simulink model "SDRE_MPTA_SDRE_newMODEL"  (R2024a)
settings: Solver=ode23t  StartTime=0  StopTime=27.8  RelTol=1e-3
values from neighbouring files (symbols this model uses):
  B = 0.002277    [initial_value.m]
  coef = readmatrix(ReadPath_coef)    [inital.m]
  command_t = readmatrix(ReadPath_command_t)    [inital.m]
  J = 0.00782    [initial_value.m]
  Lambda_m = 0.30175    [initial_value.m]
  Ld = 18e-3    (= 0.018)    [initial_value.m]
  Ldq = Ld - Lq    [inital.m]
  Lq = 32e-3    (= 0.032)    [initial_value.m]
  Polepairs = 3    [initial_value.m]
  rate1 = 3    [inital.m]
  rate2 = 1    [inital.m]
  Rs = 2.5    [initial_value.m]
  timestep = 1e-5    (= 1e-05)    [inital.m]
  V = [V_11 V_12;V_21 V_22]    [Create_MVG.m]
undefined symbols (not defined in the file or in its folder): rate
libraries: spsControlledVoltageSourceLib x6, spsPermanentMagnetSynchronousMachineLib x2, spsGroundLib x2, sps_lib x1
(part 1 of 2)
settings Model: Creator=User  LastModifiedBy=User

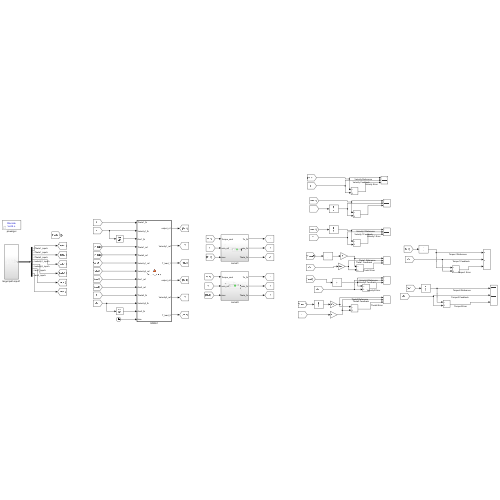
[thumbnail: Simulink's stored preview of the top-level diagram]
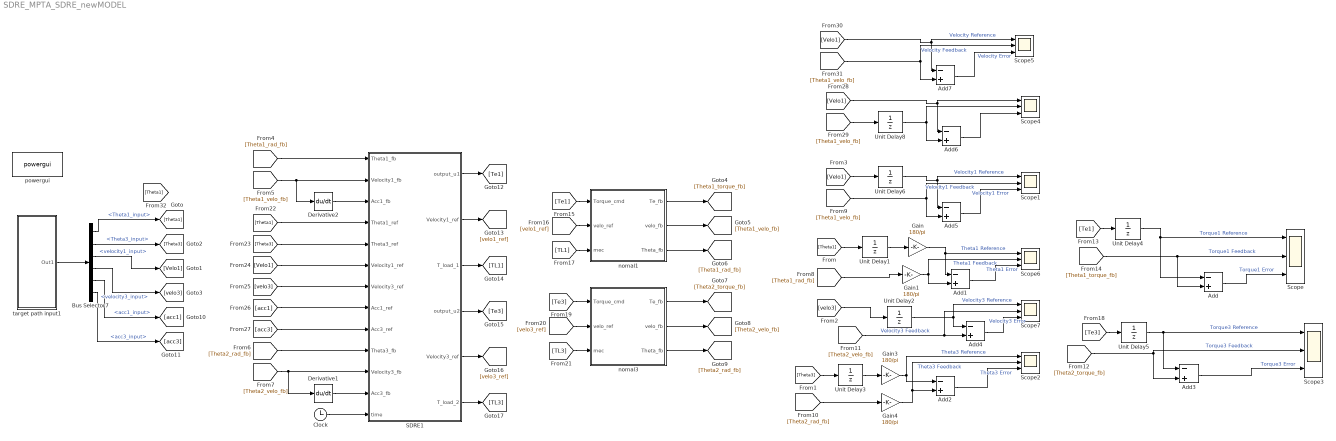
== system SDRE_MPTA_SDRE_newMODEL ==
  Add{,1..7} (8 alike) : Sum  Inputs=-+
  Bus Selector7 : BusSelector  OutputSignals=Theta1_input,Theta3_input,velocity1_input,velocity3_input,acc1_input,acc3_input
  Clock : Clock
  Derivative1 : Derivative
  Derivative2 : Derivative
  Gain{,1,3..4} (4 alike) : Gain  Gain=180/pi
  SDRE1 : MATLAB Function  TreatAsAtomicUnit=on
  Scope{,1..7} (8 alike) : Scope  NumInputPorts=3
  Unit Delay{1..6,8} (7 alike) : UnitDelay  SampleTime=1e-5  HasFrameUpgradeWarning=on
  nomal1 : Subsystem
  nomal3 : Subsystem
  powergui : sps_lib/powergui  Priority=1  SimulationMode=Discrete  SampleTime=timestep  frequency=60  Iterations=50  frequencyindice=0  Pbase=100e6  ErrMax=1e-4  UnitsV=kV  UnitsW=MW  buscounter=0  FunctionMessages=off  echomessages=off  EnableUseOfTLC=off  CurrentSourceSwitches=off  DisableSnubberDevices=off  DisableRonSwitches=off  DisableVfSwitches=off  DisplayEquations=off  AutomaticDiscreteSolvers=off  SolverType=Tustin/Backward Euler (TBE)  Interpol=off  ExternalGateDelay=off  methode=off  Ts=100  x0status=blocks  SPID=on  SwTol=0  HookPort=off  NonlinearTolerance=1e-4  nMaxIteration=100  ContinueOnMaxIteration=off  RestoreLinks=warning  ResistiveCurrentMeasurement=off  Frange=[0:2:500]  Ylog=off  Xlog=on  ShowGrid=off  save=off  variable=ZData  structure=0  ZoomFFT=off  StartTime=0.0  cycles=1  DisplayStyle=1  fundamental=60  FreqAxis=off  MaxFrequency=1000  frequencyindicesteady=1  RmsSteady=1  display=off
  target path input1 : Subsystem
  wires:
  Bus Selector7/4 -> [velo3]  "<velocity3_input>"
  Bus Selector7/2 -> [Theta3]  "<Theta3_input>"
  Bus Selector7/1 -> [Theta1]  "<Theta1_input>"
  Bus Selector7/3 -> [Velo1]  "<velocity1_input>"
  SDRE1/4(output_u2) -> [Te3]
  SDRE1/2(Velocity1_ref) -> [velo1_ref]
  [Theta3] -> Unit Delay3/1
  [velo3] -> Unit Delay2/1
  target path input1/1(Out1) -> Bus Selector7/1
  nomal1/1(Te_fb) -> [Theta1_torque_fb]
  nomal1/2(velo_fb) -> [Theta1_velo_fb]
  nomal1/3(Theta_fb) -> [Theta1_rad_fb]
  [Theta1_rad_fb] -> SDRE1/1(Theta1_fb)
  [Theta1_velo_fb] -> Derivative2/1, SDRE1/2(Velocity1_fb)
  [Theta2_rad_fb] -> SDRE1/10(Theta3_fb)
  [Theta2_velo_fb] -> Derivative1/1, SDRE1/11(Velocity3_fb)
  Gain/1 -> Add1/1, Scope6/1  "Theta1 Reference"
  Gain1/1 -> Scope6/2, Add1/2  "Theta1 Feedback"
  Gain3/1 -> Add2/1, Scope2/1  "Theta3 Reference"
  Gain4/1 -> Add2/2, Scope2/2  "Theta3 Feedback"
  Add2/1 -> Scope2/3  "Theta3 Error"
  Add1/1 -> Scope6/3  "Theta1 Error"
  Add3/1 -> Scope3/3  "Torque3 Error"
  Derivative1/1 -> SDRE1/12(Acc3_fb)
  Derivative2/1 -> SDRE1/3(Acc1_fb)
  Add/1 -> Scope/3  "Torque1 Error"
  Add4/1 -> Scope7/3  "Velocity3 Error"
  Add5/1 -> Scope1/3  "Velocity1 Error"
  Clock/1 -> SDRE1/13(time)
  SDRE1/1(output_u1) -> [Te1]
  [Theta1] -> Unit Delay1/1
  [Velo1] -> Unit Delay6/1
  [Theta2_velo_fb] -> Add4/2, Scope7/2  "Velocity3 Feedback"
  [Theta2_rad_fb] -> Gain4/1
  nomal3/3(Theta_fb) -> [Theta2_rad_fb]
  nomal3/2(velo_fb) -> [Theta2_velo_fb]
  nomal3/1(Te_fb) -> [Theta2_torque_fb]
  Bus Selector7/5 -> [acc1]  "<acc1_input>"
  Bus Selector7/6 -> [acc3]  "<acc3_input>"
  [Te1] -> Unit Delay4/1
  [Te1] -> nomal1/1(Torque_cmd)
  [velo1_ref] -> nomal1/2(velo_ref)
  SDRE1/3(T_load_1) -> [TL1]
  [TL1] -> nomal1/3(mec)
  [Te3] -> Unit Delay5/1
  SDRE1/5(Velocity3_ref) -> [velo3_ref]
  SDRE1/6(T_load_2) -> [TL3]
  [Te3] -> nomal3/1(Torque_cmd)
  [velo3_ref] -> nomal3/2(velo_ref)
  [TL3] -> nomal3/3(mec)
  [Theta1] -> SDRE1/4(Theta1_ref)
  [Theta3] -> SDRE1/5(Theta3_ref)
  [Velo1] -> SDRE1/6("Velocity1_ref ")
  [velo3] -> SDRE1/7("Velocity3_ref ")
  [acc1] -> SDRE1/8(Acc1_ref)
  [acc3] -> SDRE1/9(Acc3_ref)
  [Theta1_rad_fb] -> Gain1/1
  [Theta1_velo_fb] -> Add5/2, Scope1/2  "Velocity1 Feedback"
  [Theta1_torque_fb] -> Add/2, Scope/2  "Torque1 Feedback"
  [Theta2_torque_fb] -> Scope3/2, Add3/2  "Torque3 Feedback"
  Unit Delay6/1 -> Add5/1, Scope1/1  "Velocity1 Reference"
  Unit Delay1/1 -> Gain/1
  Unit Delay3/1 -> Gain3/1
  Unit Delay2/1 -> Scope7/1, Add4/1  "Velocity3 Reference"
  Unit Delay4/1 -> Add/1, Scope/1  "Torque1 Reference"
  Unit Delay5/1 -> Scope3/1, Add3/1  "Torque3 Reference"
  Add6/1 -> Scope4/3
  [Theta1_velo_fb] -> Unit Delay8/1
  [Velo1] -> Add6/1, Scope4/1
  Unit Delay8/1 -> Add6/2, Scope4/2
  Add7/1 -> Scope5/3  "Velocity Error"
  [Theta1_velo_fb] -> Add7/2, Scope5/2  "Velocity Feedback"
  [Velo1] -> Add7/1, Scope5/1  "Velocity Reference"

== system SDRE_MPTA_SDRE_newMODEL/nomal1 ==
  Torque_cmd : Inport
  velo_ref : Inport  Port=2
  mec : Inport  Port=3
  Constant2 : Constant  Value=Polepairs
  MTPA : MATLAB Function  TreatAsAtomicUnit=on
  Measure : Subsystem
  "Permanent Magnet Synchronous Machine " : spsPermanentMagnetSynchronousMachineLib/Permanent Magnet Synchronous Machine  NbPhases=3  FluxDistribution=Sinusoidal  RotorType=Salient-pole  MechanicalLoad=Torque Tm  PresetModel=No  ShowDetailedParameters=on  MeasurementBus=off  Resistance=Rs  Inductance=8.5e-3  dqInductances=[Ld Lq]  La=5.7e-3  MachineConstant=Flux linkage established by magnets (V.s)  Flux=Lambda_m  VoltageCst=164.1942  TorqueCst=1.3579  Flat=120  Mechanical=[J B Polepairs]  PolePairs=4  InitialConditions=[0,0, 0,0]  InitialConditions5ph=[0 0 0 0 0 0]  RefAngle=Aligned with phase A axis (original Park)  IterativeDiscreteModel=Trapezoidal non iterative  TsBlock=-1  TsPowergui=0
  Product1 : Product
  Unit Delay1 : UnitDelay  SampleTime=1e-5  HasFrameUpgradeWarning=on
  toq to voltageABC1 : Subsystem  Commented=on
  toq to voltageABC6 : Subsystem
  Te_fb : Outport
  velo_fb : Outport  Port=2
  Theta_fb : Outport  Port=3
  wires:
  Constant2/1 -> Product1/2
  Product1/1 -> toq to voltageABC6/5(Theta_e)
  mec/1 -> "Permanent Magnet Synchronous Machine "/1
  Measure/1(wm) -> velo_fb/1
  Measure/2(The) -> Theta_fb/1, Product1/1
  Measure/3(Te) -> Te_fb/1
  velo_ref/1 -> toq to voltageABC6/3(velo_ref)
  Torque_cmd/1 -> MTPA/1(Te)
  "Permanent Magnet Synchronous Machine "/1 -> Unit Delay1/1, Measure/1(m)
  Unit Delay1/1 -> toq to voltageABC6/4(fb)
  MTPA/1(id_ref) -> toq to voltageABC6/1(id_ref)
  MTPA/2(iq_ref) -> toq to voltageABC6/2(iq_ref)
  connections:
  "Permanent Magnet Synchronous Machine "/LConn1 -- toq to voltageABC6/RConn1
  "Permanent Magnet Synchronous Machine "/LConn2 -- toq to voltageABC6/RConn2
  "Permanent Magnet Synchronous Machine "/LConn3 -- toq to voltageABC6/RConn3

== system SDRE_MPTA_SDRE_newMODEL/nomal3 ==
  Torque_cmd : Inport
  velo_ref : Inport  Port=2
  mec : Inport  Port=3
  Constant2 : Constant  Value=4
  MTPA : MATLAB Function  TreatAsAtomicUnit=on
  Measure : Subsystem
  "Permanent Magnet Synchronous Machine " : spsPermanentMagnetSynchronousMachineLib/Permanent Magnet Synchronous Machine  NbPhases=3  FluxDistribution=Sinusoidal  RotorType=Salient-pole  MechanicalLoad=Torque Tm  PresetModel=No  ShowDetailedParameters=on  MeasurementBus=off  Resistance=Rs  Inductance=8.5e-3  dqInductances=[Ld Lq]  La=5.7e-3  MachineConstant=Flux linkage established by magnets (V.s)  Flux=Lambda_m  VoltageCst=164.1942  TorqueCst=1.3579  Flat=120  Mechanical=[J B Polepairs]  PolePairs=4  InitialConditions=[0,0, 0,0]  InitialConditions5ph=[0 0 0 0 0 0]  RefAngle=Aligned with phase A axis (original Park)  IterativeDiscreteModel=Trapezoidal non iterative  TsBlock=-1  TsPowergui=0
  Product1 : Product
  Scope : Scope  NumInputPorts=2
  Scope1 : Scope
  Scope3 : Scope  NumInputPorts=2
  Unit Delay1 : UnitDelay  SampleTime=1e-5  HasFrameUpgradeWarning=on
  toq to voltageABC : Subsystem
  toq to voltageABC6 : Subsystem
  Te_fb : Outport
  velo_fb : Outport  Port=2
  Theta_fb : Outport  Port=3
  wires:
  Measure/4(Vs_q) -> Scope/1
  Measure/5(Vs_d) -> Scope/2
  Constant2/1 -> Product1/2
  Product1/1 -> Scope1/1, toq to voltageABC6/5(Theta_e)
  mec/1 -> "Permanent Magnet Synchronous Machine "/1, Scope3/1
  Measure/1(wm) -> velo_fb/1
  Measure/2(The) -> Theta_fb/1, Product1/1
  Measure/3(Te) -> Te_fb/1
  velo_ref/1 -> toq to voltageABC6/3(velo_ref)
  Torque_cmd/1 -> Scope3/2, MTPA/1(Te), toq to voltageABC/1(Tref)
  "Permanent Magnet Synchronous Machine "/1 -> Unit Delay1/1, Measure/1(m)
  Unit Delay1/1 -> toq to voltageABC6/4(fb)
  MTPA/1(id_ref) -> toq to voltageABC6/1(id_ref)
  MTPA/2(iq_ref) -> toq to voltageABC6/2(iq_ref)
  connections:
  "Permanent Magnet Synchronous Machine "/LConn1 -- toq to voltageABC6/RConn1
  "Permanent Magnet Synchronous Machine "/LConn2 -- toq to voltageABC6/RConn2
  "Permanent Magnet Synchronous Machine "/LConn3 -- toq to voltageABC6/RConn3

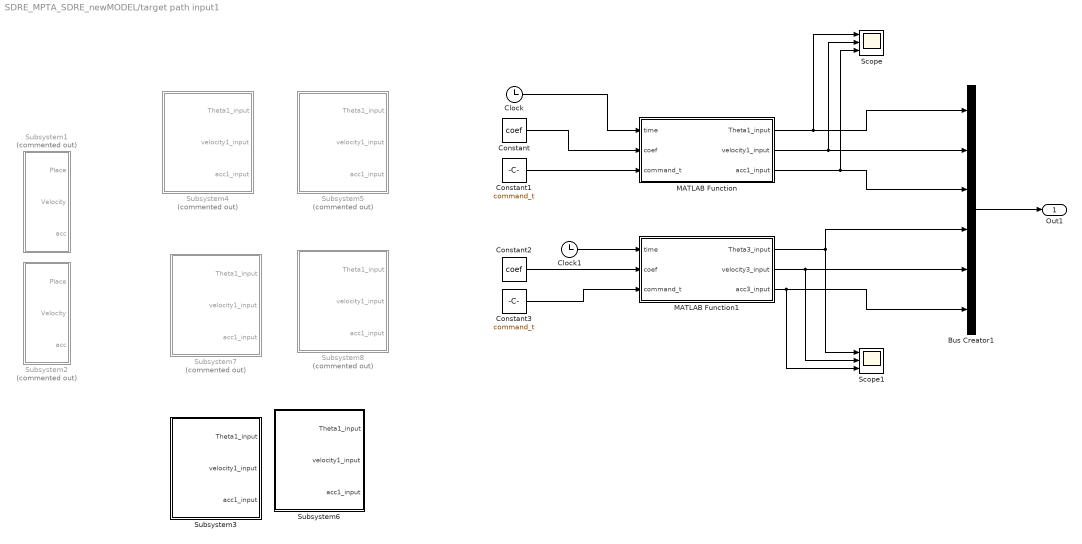
== system SDRE_MPTA_SDRE_newMODEL/target path input1 ==
  Bus Creator1 : BusCreator  Inputs=6
  Clock : Clock
  Clock1 : Clock
  Constant : Constant  Value=coef
  Constant1 : Constant  Value=command_t
  Constant2 : Constant  Value=coef
  Constant3 : Constant  Value=command_t
  MATLAB Function : MATLAB Function  TreatAsAtomicUnit=on
  MATLAB Function1 : MATLAB Function  TreatAsAtomicUnit=on
  Scope : Scope  NumInputPorts=3
  Scope1 : Scope  NumInputPorts=3
  Subsystem1 : Subsystem  Commented=on
  Subsystem2 : Subsystem  Commented=on
  Subsystem3 : Subsystem
  Subsystem4 : Subsystem  Commented=on
  Subsystem5 : Subsystem  Commented=on
  Subsystem6 : Subsystem
  Subsystem7 : Subsystem  Commented=on
  Subsystem8 : Subsystem  Commented=on
  Out1 : Outport
  wires:
  Bus Creator1/1 -> Out1/1
  Clock/1 -> MATLAB Function/1(time)
  Constant/1 -> MATLAB Function/2(coef)
  Constant1/1 -> MATLAB Function/3(command_t)
  Clock1/1 -> MATLAB Function1/1(time)
  Constant3/1 -> MATLAB Function1/3(command_t)
  Constant2/1 -> MATLAB Function1/2(coef)
  MATLAB Function/1(Theta1_input) -> Scope/1, Bus Creator1/1
  MATLAB Function/2(velocity1_input) -> Scope/2, Bus Creator1/2
  MATLAB Function/3(acc1_input) -> Scope/3, Bus Creator1/3
  MATLAB Function1/1(Theta3_input) -> Bus Creator1/4, Scope1/1
  MATLAB Function1/2(velocity3_input) -> Bus Creator1/5, Scope1/2
  MATLAB Function1/3(acc3_input) -> Bus Creator1/6, Scope1/3

== system SDRE_MPTA_SDRE_newMODEL/nomal1/Measure ==
  m : Inport
  Bus Selector1 : BusSelector  OutputSignals=Rotor speed wm (rad/s),Rotor angle thetam (rad),Electromagnetic torque Te (N*m),Stator voltage Vs_q (V),Stator voltage Vs_d (V)
  Rate_Transition{1..5} (5 alike) : RateTransition  Integrity=off
  wm : Outport
  The : Outport  Port=2
  Te : Outport  Port=3
  Vs_q : Outport  Port=4
  Vs_d : Outport  Port=5
  wires:
  Bus Selector1/5 -> Rate_Transition5/1  "<Stator voltage Vs_d (V)>"
  Bus Selector1/4 -> Rate_Transition4/1  "<Stator voltage Vs_q (V)>"
  Bus Selector1/1 -> Rate_Transition1/1  "<Rotor speed wm (rad/s)>"
  m/1 -> Bus Selector1/1
  Bus Selector1/3 -> Rate_Transition3/1  "<Electromagnetic torque Te (N*m)>"
  Bus Selector1/2 -> Rate_Transition2/1  "<Rotor angle thetam (rad)>"
  Rate_Transition1/1 -> wm/1
  Rate_Transition2/1 -> The/1
  Rate_Transition3/1 -> Te/1
  Rate_Transition4/1 -> Vs_q/1
  Rate_Transition5/1 -> Vs_d/1

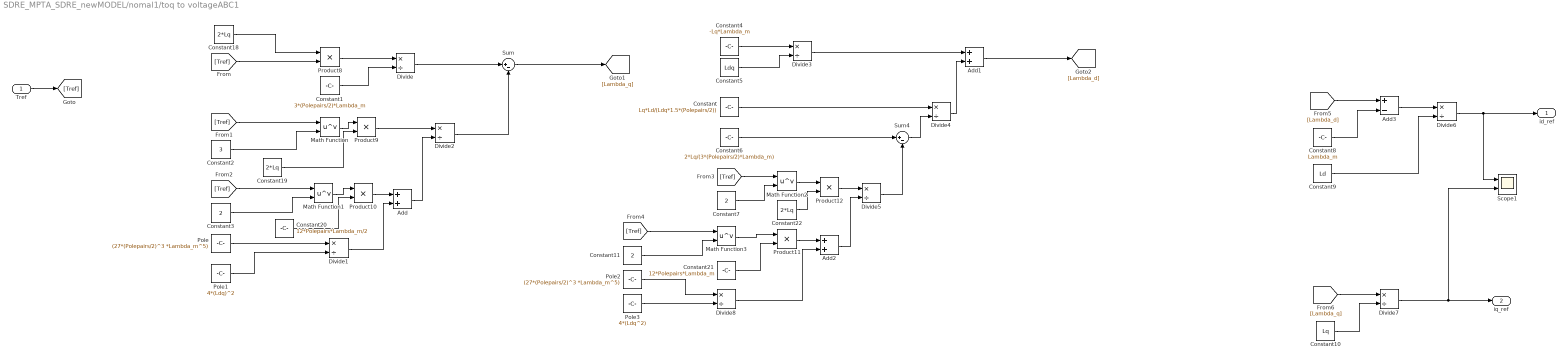
== system SDRE_MPTA_SDRE_newMODEL/nomal1/toq to voltageABC1 ==
  Tref : Inport
  Add : Sum
  Add1 : Sum
  Add2 : Sum
  Add3 : Sum  Inputs=+-
  Constant : Constant  Value=Lq*Ld/(Ldq*1.5*(Polepairs/2))
  Constant1 : Constant  Value=3*(Polepairs/2)*Lambda_m
  Constant10 : Constant  Value=Lq
  Constant11 : Constant  Value=2
  Constant18 : Constant  Value=2*Lq
  Constant19 : Constant  Value=2*Lq
  Constant2 : Constant  Value=3
  Constant20 : Constant  Value=12*Polepairs*Lambda_m/2
  Constant21 : Constant  Value=12*Polepairs*Lambda_m
  Constant22 : Constant  Value=2*Lq
  Constant3 : Constant  Value=2
  Constant4 : Constant  Value=-Lq*Lambda_m
  Constant5 : Constant  Value=Ldq
  Constant6 : Constant  Value=2*Lq/(3*(Polepairs/2)*Lambda_m)
  Constant7 : Constant  Value=2
  Constant8 : Constant  Value=Lambda_m
  Constant9 : Constant  Value=Ld
  Divide{,1..8} (9 alike) : Product  Inputs=*/
  Math Function{,1..3} (4 alike) : Math  Operator=pow
  Pole : Constant  Value=(27*(Polepairs/2)^3 *Lambda_m^5)
  Pole1 : Constant  Value=4*(Ldq)^2
  Pole2 : Constant  Value=(27*(Polepairs/2)^3 *Lambda_m^5)
  Pole3 : Constant  Value=4*(Ldq^2)
  Product{8..12} (5 alike) : Product
  Scope1 : Scope  NumInputPorts=2
  Sum : Sum  Inputs=|+-
  Sum4 : Sum  Inputs=|+-
  id_ref : Outport
  iq_ref : Outport  Port=2
  wires:
  Tref/1 -> [Tref]
  [Tref] -> Product8/2
  Product8/1 -> Divide/1
  Constant1/1 -> Divide/2
  [Tref] -> Math Function/1
  Constant2/1 -> Math Function/2
  [Tref] -> Math Function1/1
  Constant3/1 -> Math Function1/2
  Product10/1 -> Add/1
  Pole/1 -> Divide1/1
  Pole1/1 -> Divide1/2
  Divide1/1 -> Add/2
  Add/1 -> Divide2/2
  Product9/1 -> Divide2/1
  Divide/1 -> Sum/1
  Divide2/1 -> Sum/2
  Constant4/1 -> Divide3/1
  Constant5/1 -> Divide3/2
  Divide3/1 -> Add1/1
  Constant/1 -> Divide4/1
  Constant6/1 -> Sum4/1
  [Tref] -> Math Function2/1
  Constant7/1 -> Math Function2/2
  Product12/1 -> Divide5/1
  Sum4/1 -> Divide4/2
  Divide5/1 -> Sum4/2
  Divide4/1 -> Add1/2
  Pole2/1 -> Divide8/1
  [Tref] -> Math Function3/1
  Pole3/1 -> Divide8/2
  Divide8/1 -> Add2/2
  Constant11/1 -> Math Function3/2
  Product11/1 -> Add2/1
  Add2/1 -> Divide5/2
  Constant18/1 -> Product8/1
  Math Function/1 -> Product9/1
  Constant19/1 -> Product9/2
  Math Function1/1 -> Product10/1
  Constant20/1 -> Product10/2
  Math Function3/1 -> Product11/1
  Constant21/1 -> Product11/2
  Math Function2/1 -> Product12/1
  Constant22/1 -> Product12/2
  Sum/1 -> [Lambda_q]
  [Lambda_d] -> Add3/1
  Constant8/1 -> Add3/2
  Add3/1 -> Divide6/1
  Constant9/1 -> Divide6/2
  Divide6/1 -> Scope1/1, id_ref/1
  [Lambda_q] -> Divide7/1
  Constant10/1 -> Divide7/2
  Divide7/1 -> Scope1/2, iq_ref/1
  Add1/1 -> [Lambda_d]

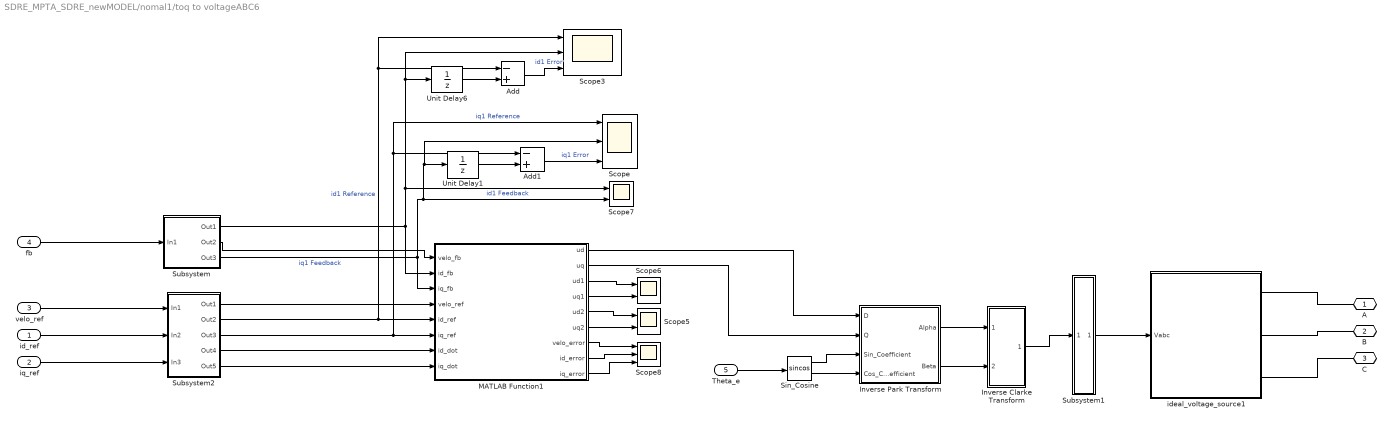
== system SDRE_MPTA_SDRE_newMODEL/nomal1/toq to voltageABC6 ==
  id_ref : Inport
  iq_ref : Inport  Port=2
  velo_ref : Inport  Port=3
  fb : Inport  Port=4
  Theta_e : Inport  Port=5
  Add : Sum  Inputs=-+
  Add1 : Sum  Inputs=-+
  Inverse Clarke Transform : Subsystem
  Inverse Park Transform : Subsystem
  MATLAB Function1 : MATLAB Function  TreatAsAtomicUnit=on
  Scope : Scope  NumInputPorts=3
  Scope3 : Scope  NumInputPorts=3
  Scope5 : Scope  NumInputPorts=2
  Scope6 : Scope  NumInputPorts=2
  Scope7 : Scope  NumInputPorts=2
  Scope8 : Scope  NumInputPorts=3
  Sin_Cosine : Trigonometry  Operator=sincos
  Subsystem : Subsystem
  Subsystem1 : Subsystem
      mask Display: fprintf('D/C')
  Subsystem2 : Subsystem
  Unit Delay1 : UnitDelay  SampleTime=1e-5  HasFrameUpgradeWarning=on
  Unit Delay6 : UnitDelay  SampleTime=1e-5  HasFrameUpgradeWarning=on
  ideal_voltage_source1 : Subsystem  VariantControl=variantPwm == enumPwm.behavior
  A : PMIOPort  Side=Right
  B : PMIOPort  Port=2  Side=Right
  C : PMIOPort  Port=3  Side=Right
  wires:
  MATLAB Function1/5(ud2) -> Scope5/1
  MATLAB Function1/6(uq2) -> Scope5/2
  MATLAB Function1/3(ud1) -> Scope6/1
  MATLAB Function1/4(uq1) -> Scope6/2
  MATLAB Function1/7(velo_error) -> Scope8/1
  MATLAB Function1/8(id_error) -> Scope8/2
  MATLAB Function1/9(iq_error) -> Scope8/3
  Add/1 -> Scope3/3  "id1 Error"
  Add1/1 -> Scope/3  "iq1 Error"
  MATLAB Function1/1(ud) -> Inverse Park Transform/1(D)
  MATLAB Function1/2(uq) -> Inverse Park Transform/2(Q)
  Theta_e/1 -> Sin_Cosine/1
  Sin_Cosine/1 -> Inverse Park Transform/3(Sin_Coefficient)
  Sin_Cosine/2 -> Inverse Park Transform/4(Cos_Coefficient)
  Inverse Park Transform/1(Alpha) -> Inverse Clarke Transform/1(Alpha)
  Inverse Park Transform/2(Beta) -> Inverse Clarke Transform/2(Beta)
  Inverse Clarke Transform/1(ABC) -> Subsystem1/1(In1)
  Subsystem1/1(Out1) -> ideal_voltage_source1/1(Vabc)
  Subsystem/3(Out3) -> MATLAB Function1/3(iq_fb), Scope7/2, Scope/2, Unit Delay1/1  "iq1 Feedback"
  Subsystem/2(Out2) -> MATLAB Function1/1(velo_fb)
  fb/1 -> Subsystem/1(In1)
  Subsystem2/3(Out3) -> Scope/1, Add1/1, MATLAB Function1/6(iq_ref)  "iq1 Reference"
  Subsystem2/2(Out2) -> Scope3/1, Add/1, MATLAB Function1/5(id_ref)  "id1 Reference"
  Subsystem2/1(Out1) -> MATLAB Function1/4(velo_ref)
  Subsystem2/4(Out4) -> MATLAB Function1/7(id_dot)
  Subsystem2/5(Out5) -> MATLAB Function1/8(iq_dot)
  velo_ref/1 -> Subsystem2/1(In1)
  id_ref/1 -> Subsystem2/2(In2)
  iq_ref/1 -> Subsystem2/3(In3)
  Subsystem/1(Out1) -> Scope7/1, Unit Delay6/1, Scope3/2, MATLAB Function1/2(id_fb)  "id1 Feedback"
  Unit Delay6/1 -> Add/2
  Unit Delay1/1 -> Add1/2
  connections:
  ideal_voltage_source1/RConn1 -- A/RConn1
  ideal_voltage_source1/RConn2 -- B/RConn1
  ideal_voltage_source1/RConn3 -- C/RConn1

== system SDRE_MPTA_SDRE_newMODEL/nomal3/Measure ==
  m : Inport
  Bus Selector1 : BusSelector  OutputSignals=Rotor speed wm (rad/s),Rotor angle thetam (rad),Electromagnetic torque Te (N*m),Stator voltage Vs_q (V),Stator voltage Vs_d (V)
  Rate_Transition{1..5} (5 alike) : RateTransition  Integrity=off
  wm : Outport
  The : Outport  Port=2
  Te : Outport  Port=3
  Vs_q : Outport  Port=4
  Vs_d : Outport  Port=5
  wires:
  Bus Selector1/5 -> Rate_Transition5/1  "<Stator voltage Vs_d (V)>"
  Bus Selector1/4 -> Rate_Transition4/1  "<Stator voltage Vs_q (V)>"
  Bus Selector1/1 -> Rate_Transition1/1  "<Rotor speed wm (rad/s)>"
  m/1 -> Bus Selector1/1
  Bus Selector1/3 -> Rate_Transition3/1  "<Electromagnetic torque Te (N*m)>"
  Bus Selector1/2 -> Rate_Transition2/1  "<Rotor angle thetam (rad)>"
  Rate_Transition1/1 -> wm/1
  Rate_Transition2/1 -> The/1
  Rate_Transition3/1 -> Te/1
  Rate_Transition4/1 -> Vs_q/1
  Rate_Transition5/1 -> Vs_d/1

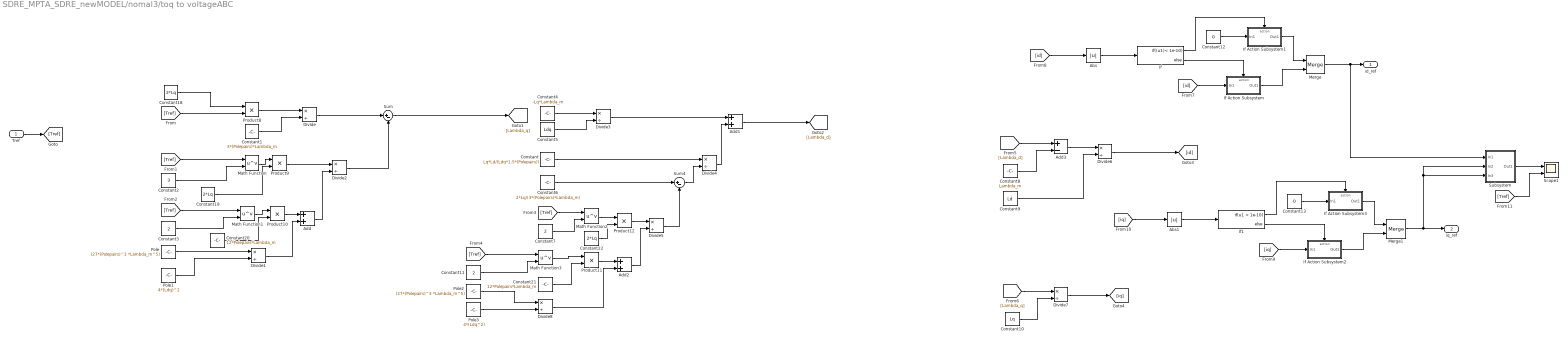
== system SDRE_MPTA_SDRE_newMODEL/nomal3/toq to voltageABC ==
  Tref : Inport
  Abs : Abs  SaturateOnIntegerOverflow=off
  Abs1 : Abs  SaturateOnIntegerOverflow=off
  Add : Sum
  Add1 : Sum
  Add2 : Sum
  Add3 : Sum  Inputs=+-
  Constant : Constant  Value=Lq*Ld/(Ldq*1.5*(Polepairs))
  Constant1 : Constant  Value=3*(Polepairs)*Lambda_m
  Constant10 : Constant  Value=Lq
  Constant11 : Constant  Value=2
  Constant12 : Constant  Value=0
  Constant13 : Constant  Value=0
  Constant18 : Constant  Value=2*Lq
  Constant19 : Constant  Value=2*Lq
  Constant2 : Constant  Value=3
  Constant20 : Constant  Value=12*Polepairs*Lambda_m
  Constant21 : Constant  Value=12*Polepairs*Lambda_m
  Constant22 : Constant  Value=2*Lq
  Constant3 : Constant  Value=2
  Constant4 : Constant  Value=-Lq*Lambda_m
  Constant5 : Constant  Value=Ldq
  Constant6 : Constant  Value=2*Lq/(3*(Polepairs)*Lambda_m)
  Constant7 : Constant  Value=2
  Constant8 : Constant  Value=Lambda_m
  Constant9 : Constant  Value=Ld
  Divide{,1..8} (9 alike) : Product  Inputs=*/
  If : If  IfExpression=(u1)< 1e-10
  If Action Subsystem : Subsystem  TreatAsAtomicUnit=on
  If Action Subsystem1 : Subsystem  TreatAsAtomicUnit=on
  If Action Subsystem2 : Subsystem  TreatAsAtomicUnit=on
  If Action Subsystem3 : Subsystem  TreatAsAtomicUnit=on
  If1 : If  IfExpression=u1 < 1e-10
  Math Function{,1..3} (4 alike) : Math  Operator=pow
  Merge : Merge
  Merge1 : Merge
  Pole : Constant  Value=(27*(Polepairs)^3 *Lambda_m^5)
  Pole1 : Constant  Value=4*(Ldq)^2
  Pole2 : Constant  Value=(27*(Polepairs)^3 *Lambda_m^5)
  Pole3 : Constant  Value=4*(Ldq^2)
  Product{8..12} (5 alike) : Product
  Scope1 : Scope  NumInputPorts=2
  Subsystem : Subsystem
  Sum : Sum  Inputs=|+-
  Sum4 : Sum  Inputs=|+-
  id_ref : Outport
  iq_ref : Outport  Port=2
  wires:
  Tref/1 -> [Tref]
  [Tref] -> Product8/2
  Product8/1 -> Divide/1
  Constant1/1 -> Divide/2
  [Tref] -> Math Function/1
  Constant2/1 -> Math Function/2
  [Tref] -> Math Function1/1
  Constant3/1 -> Math Function1/2
  Product10/1 -> Add/1
  Pole/1 -> Divide1/1
  Pole1/1 -> Divide1/2
  Divide1/1 -> Add/2
  Add/1 -> Divide2/2
  Product9/1 -> Divide2/1
  Divide/1 -> Sum/1
  Divide2/1 -> Sum/2
  Constant18/1 -> Product8/1
  Math Function/1 -> Product9/1
  Constant19/1 -> Product9/2
  Math Function1/1 -> Product10/1
  Constant20/1 -> Product10/2
  Sum/1 -> [Lambda_q]
  [Lambda_d] -> Add3/1
  Constant8/1 -> Add3/2
  Add3/1 -> Divide6/1
  Constant9/1 -> Divide6/2
  Divide6/1 -> [id]
  [Lambda_q] -> Divide7/1
  Constant10/1 -> Divide7/2
  Pole2/1 -> Divide8/1
  Constant7/1 -> Math Function2/2
  Add1/1 -> [Lambda_d]
  Divide3/1 -> Add1/1
  Constant4/1 -> Divide3/1
  Product12/1 -> Divide5/1
  Constant22/1 -> Product12/2
  Constant21/1 -> Product11/2
  Math Function3/1 -> Product11/1
  Math Function2/1 -> Product12/1
  Product11/1 -> Add2/1
  Constant/1 -> Divide4/1
  [Tref] -> Math Function2/1
  Divide4/1 -> Add1/2
  Sum4/1 -> Divide4/2
  Constant11/1 -> Math Function3/2
  Constant6/1 -> Sum4/1
  Pole3/1 -> Divide8/2
  Add2/1 -> Divide5/2
  Divide8/1 -> Add2/2
  [Tref] -> Math Function3/1
  Constant5/1 -> Divide3/2
  Divide5/1 -> Sum4/2
  If/2 -> If Action Subsystem/Action
  If/1 -> If Action Subsystem1/Action
  Constant12/1 -> If Action Subsystem1/1(In1)
  If Action Subsystem1/1(Out1) -> Merge/1
  If Action Subsystem/1(Out1) -> Merge/2
  Merge/1 -> Subsystem/1(In1), id_ref/1
  [id] -> If Action Subsystem/1(In1)
  Divide7/1 -> [iq]
  [id] -> Abs/1
  If Action Subsystem2/1(Out1) -> Merge1/2
  [iq] -> If Action Subsystem2/1(In1)
  If Action Subsystem3/1(Out1) -> Merge1/1
  If1/2 -> If Action Subsystem2/Action
  Merge1/1 -> Subsystem/3(In3), Subsystem/2(In2), iq_ref/1
  If1/1 -> If Action Subsystem3/Action
  Constant13/1 -> If Action Subsystem3/1(In1)
  [iq] -> Abs1/1
  Abs/1 -> If/1
  Abs1/1 -> If1/1
  Subsystem/1(Out1) -> Scope1/1
  [Tref] -> Scope1/2

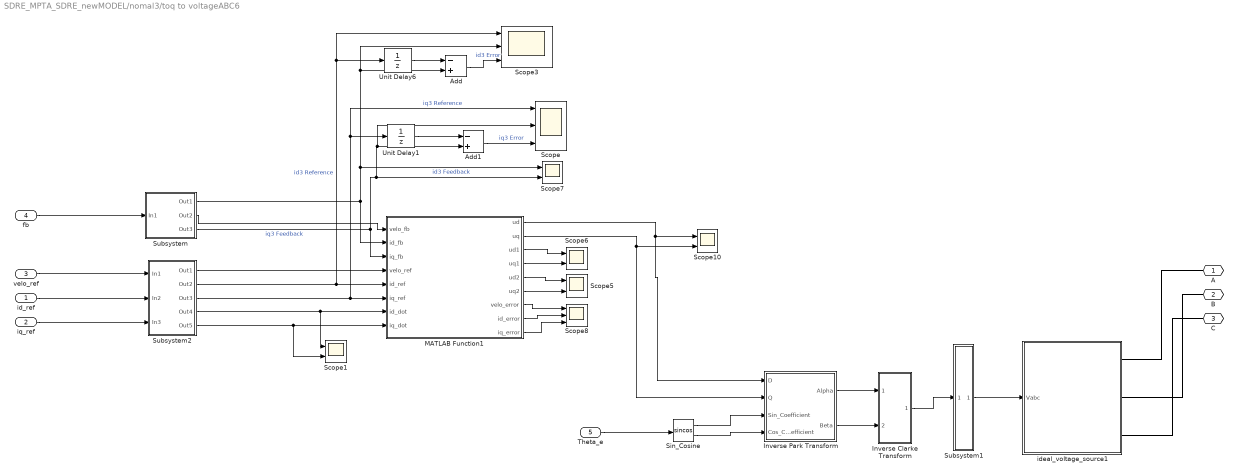
== system SDRE_MPTA_SDRE_newMODEL/nomal3/toq to voltageABC6 ==
  id_ref : Inport
  iq_ref : Inport  Port=2
  velo_ref : Inport  Port=3
  fb : Inport  Port=4
  Theta_e : Inport  Port=5
  Add : Sum  Inputs=-+
  Add1 : Sum  Inputs=-+
  Inverse Clarke Transform : Subsystem
  Inverse Park Transform : Subsystem
  MATLAB Function1 : MATLAB Function  TreatAsAtomicUnit=on
  Scope : Scope  NumInputPorts=3
  Scope{1,5..7,10} (5 alike) : Scope  NumInputPorts=2
  Scope3 : Scope  NumInputPorts=3
  Scope8 : Scope  NumInputPorts=3
  Sin_Cosine : Trigonometry  Operator=sincos
  Subsystem : Subsystem
  Subsystem1 : Subsystem
      mask Display: fprintf('D/C')
  Subsystem2 : Subsystem
  Unit Delay1 : UnitDelay  SampleTime=1e-5  HasFrameUpgradeWarning=on
  Unit Delay6 : UnitDelay  SampleTime=1e-5  HasFrameUpgradeWarning=on
  ideal_voltage_source1 : Subsystem  VariantControl=variantPwm == enumPwm.behavior
  A : PMIOPort  Side=Right
  B : PMIOPort  Port=2  Side=Right
  C : PMIOPort  Port=3  Side=Right
  wires:
  MATLAB Function1/5(ud2) -> Scope5/1
  MATLAB Function1/6(uq2) -> Scope5/2
  MATLAB Function1/3(ud1) -> Scope6/1
  MATLAB Function1/4(uq1) -> Scope6/2
  MATLAB Function1/7(velo_error) -> Scope8/1
  MATLAB Function1/8(id_error) -> Scope8/2
  MATLAB Function1/9(iq_error) -> Scope8/3
  Add/1 -> Scope3/3  "id3 Error"
  Add1/1 -> Scope/3  "iq3 Error"
  MATLAB Function1/1(ud) -> Scope10/1, Inverse Park Transform/1(D)
  MATLAB Function1/2(uq) -> Inverse Park Transform/2(Q), Scope10/2
  Theta_e/1 -> Sin_Cosine/1
  Sin_Cosine/1 -> Inverse Park Transform/3(Sin_Coefficient)
  Sin_Cosine/2 -> Inverse Park Transform/4(Cos_Coefficient)
  Inverse Park Transform/1(Alpha) -> Inverse Clarke Transform/1(Alpha)
  Inverse Park Transform/2(Beta) -> Inverse Clarke Transform/2(Beta)
  Inverse Clarke Transform/1(ABC) -> Subsystem1/1(In1)
  Subsystem1/1(Out1) -> ideal_voltage_source1/1(Vabc)
  Subsystem/2(Out2) -> MATLAB Function1/1(velo_fb)
  fb/1 -> Subsystem/1(In1)
  Subsystem2/3(Out3) -> Scope/1, Unit Delay1/1, MATLAB Function1/6(iq_ref)  "iq3 Reference"
  Subsystem2/2(Out2) -> Scope3/1, Unit Delay6/1, MATLAB Function1/5(id_ref)  "id3 Reference"
  Subsystem2/1(Out1) -> MATLAB Function1/4(velo_ref)
  Subsystem2/4(Out4) -> Scope1/1, MATLAB Function1/7(id_dot)
  Subsystem2/5(Out5) -> Scope1/2, MATLAB Function1/8(iq_dot)
  velo_ref/1 -> Subsystem2/1(In1)
  id_ref/1 -> Subsystem2/2(In2)
  iq_ref/1 -> Subsystem2/3(In3)
  Subsystem/1(Out1) -> Scope7/1, Add/2, Scope3/2, MATLAB Function1/2(id_fb)  "id3 Feedback"
  Subsystem/3(Out3) -> MATLAB Function1/3(iq_fb), Scope7/2, Add1/2, Scope/2  "iq3 Feedback"
  Unit Delay6/1 -> Add/1
  Unit Delay1/1 -> Add1/1
  connections:
  ideal_voltage_source1/RConn1 -- A/RConn1
  ideal_voltage_source1/RConn2 -- B/RConn1
  ideal_voltage_source1/RConn3 -- C/RConn1

== system SDRE_MPTA_SDRE_newMODEL/target path input1/Subsystem1 ==
  Clock : Clock
  Path function : MATLAB Function  TreatAsAtomicUnit=on
  Place : Outport
  Velocity : Outport  Port=2
  acc : Outport  Port=3
  wires:
  Clock/1 -> Path function/1(time)
  Path function/1(Place) -> Place/1  "acc"
  Path function/2(Velocity) -> Velocity/1
  Path function/3(Acc) -> acc/1

== system SDRE_MPTA_SDRE_newMODEL/target path input1/Subsystem2 ==
  Clock : Clock
  Path function : MATLAB Function  TreatAsAtomicUnit=on
  Place : Outport
  Velocity : Outport  Port=2
  acc : Outport  Port=3
  wires:
  Path function/3(Acc) -> acc/1
  Path function/2(Velocity) -> Velocity/1
  Path function/1(Place) -> Place/1  "acc"
  Clock/1 -> Path function/1(time)

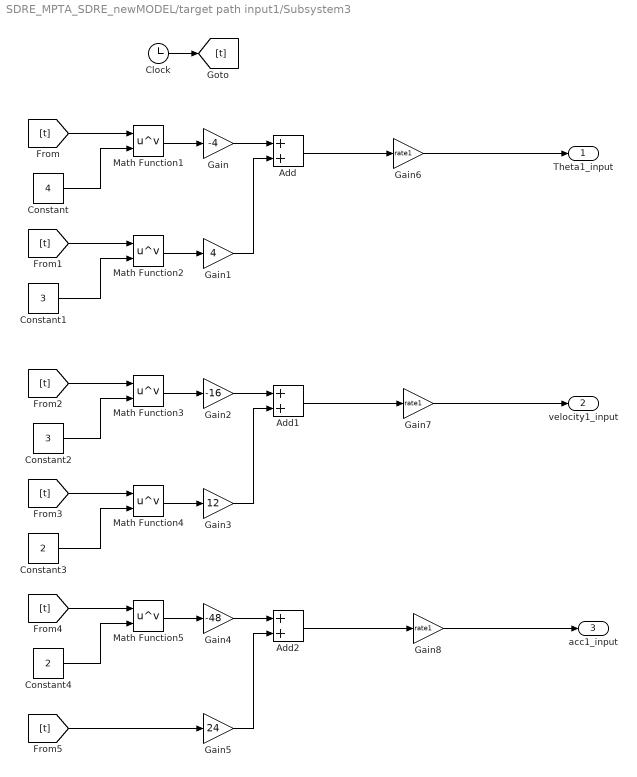
== system SDRE_MPTA_SDRE_newMODEL/target path input1/Subsystem3 ==
  Add : Sum
  Add1 : Sum
  Add2 : Sum
  Clock : Clock
  Constant : Constant  Value=4
  Constant1 : Constant  Value=3
  Constant2 : Constant  Value=3
  Constant3 : Constant  Value=2
  Constant4 : Constant  Value=2
  Gain : Gain  Gain=-4
  Gain1 : Gain  Gain=4
  Gain2 : Gain  Gain=-16
  Gain3 : Gain  Gain=12
  Gain4 : Gain  Gain=-48
  Gain5 : Gain  Gain=24
  Gain6 : Gain  Gain=rate1
  Gain7 : Gain  Gain=rate1
  Gain8 : Gain  Gain=rate1
  Math Function{1..5} (5 alike) : Math  Operator=pow
  Theta1_input : Outport
  velocity1_input : Outport  Port=2
  acc1_input : Outport  Port=3
  wires:
  Clock/1 -> [t]
  [t] -> Math Function1/1
  Constant/1 -> Math Function1/2
  Math Function1/1 -> Gain/1
  Gain/1 -> Add/1
  Gain1/1 -> Add/2
  Constant1/1 -> Math Function2/2
  [t] -> Math Function2/1
  Math Function2/1 -> Gain1/1
  Add/1 -> Gain6/1
  Gain2/1 -> Add1/1
  [t] -> Math Function4/1
  Math Function4/1 -> Gain3/1
  Gain3/1 -> Add1/2
  Constant3/1 -> Math Function4/2
  Constant2/1 -> Math Function3/2
  [t] -> Math Function3/1
  Math Function3/1 -> Gain2/1
  Add1/1 -> Gain7/1
  Gain4/1 -> Add2/1
  Gain5/1 -> Add2/2
  Constant4/1 -> Math Function5/2
  [t] -> Math Function5/1
  Math Function5/1 -> Gain4/1
  [t] -> Gain5/1
  Add2/1 -> Gain8/1
  Gain6/1 -> Theta1_input/1
  Gain7/1 -> velocity1_input/1
  Gain8/1 -> acc1_input/1

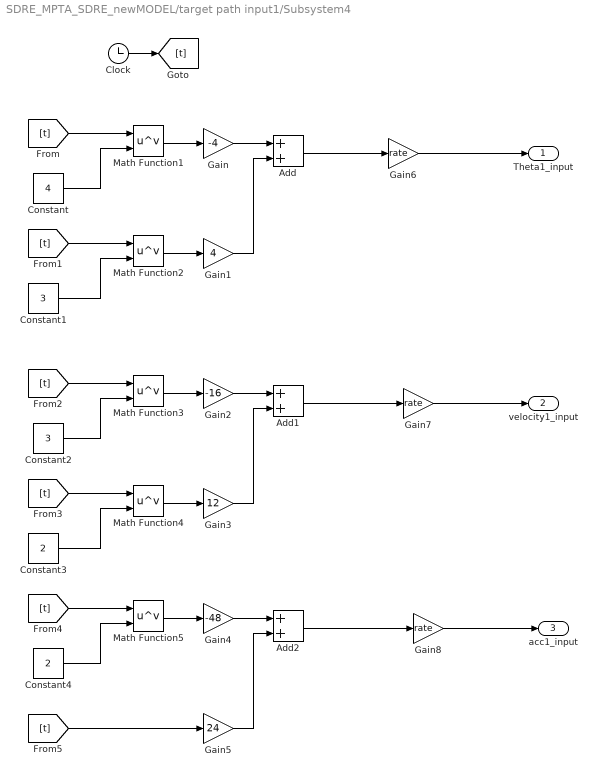
== system SDRE_MPTA_SDRE_newMODEL/target path input1/Subsystem4 ==
  Add : Sum
  Add1 : Sum
  Add2 : Sum
  Clock : Clock
  Constant : Constant  Value=4
  Constant1 : Constant  Value=3
  Constant2 : Constant  Value=3
  Constant3 : Constant  Value=2
  Constant4 : Constant  Value=2
  Gain : Gain  Gain=-4
  Gain1 : Gain  Gain=4
  Gain2 : Gain  Gain=-16
  Gain3 : Gain  Gain=12
  Gain4 : Gain  Gain=-48
  Gain5 : Gain  Gain=24
  Gain6 : Gain  Gain=rate
  Gain7 : Gain  Gain=rate
  Gain8 : Gain  Gain=rate
  Math Function{1..5} (5 alike) : Math  Operator=pow
  Theta1_input : Outport
  velocity1_input : Outport  Port=2
  acc1_input : Outport  Port=3
  wires:
  Clock/1 -> [t]
  [t] -> Math Function1/1
  Constant/1 -> Math Function1/2
  Math Function1/1 -> Gain/1
  Gain/1 -> Add/1
  Gain1/1 -> Add/2
  Constant1/1 -> Math Function2/2
  [t] -> Math Function2/1
  Math Function2/1 -> Gain1/1
  Add/1 -> Gain6/1
  Gain2/1 -> Add1/1
  [t] -> Math Function4/1
  Math Function4/1 -> Gain3/1
  Gain3/1 -> Add1/2
  Constant3/1 -> Math Function4/2
  Constant2/1 -> Math Function3/2
  [t] -> Math Function3/1
  Math Function3/1 -> Gain2/1
  Add1/1 -> Gain7/1
  Gain4/1 -> Add2/1
  Gain5/1 -> Add2/2
  Constant4/1 -> Math Function5/2
  [t] -> Math Function5/1
  Math Function5/1 -> Gain4/1
  [t] -> Gain5/1
  Add2/1 -> Gain8/1
  Gain8/1 -> acc1_input/1
  Gain7/1 -> velocity1_input/1
  Gain6/1 -> Theta1_input/1

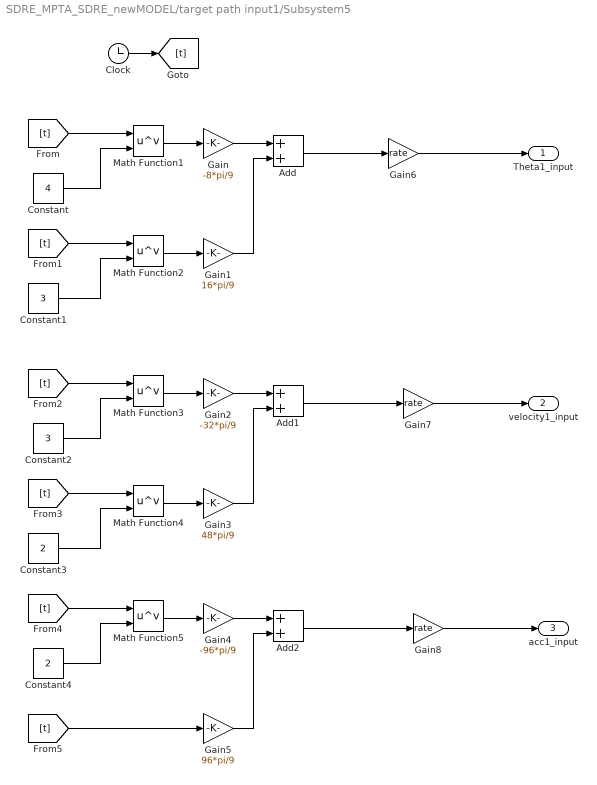
== system SDRE_MPTA_SDRE_newMODEL/target path input1/Subsystem5 ==
  Add : Sum
  Add1 : Sum
  Add2 : Sum
  Clock : Clock
  Constant : Constant  Value=4
  Constant1 : Constant  Value=3
  Constant2 : Constant  Value=3
  Constant3 : Constant  Value=2
  Constant4 : Constant  Value=2
  Gain : Gain  Gain=-8*pi/9
  Gain1 : Gain  Gain=16*pi/9
  Gain2 : Gain  Gain=-32*pi/9
  Gain3 : Gain  Gain=48*pi/9
  Gain4 : Gain  Gain=-96*pi/9
  Gain5 : Gain  Gain=96*pi/9
  Gain6 : Gain  Gain=rate
  Gain7 : Gain  Gain=rate
  Gain8 : Gain  Gain=rate
  Math Function{1..5} (5 alike) : Math  Operator=pow
  Theta1_input : Outport
  velocity1_input : Outport  Port=2
  acc1_input : Outport  Port=3
  wires:
  Clock/1 -> [t]
  [t] -> Math Function1/1
  Constant/1 -> Math Function1/2
  Math Function1/1 -> Gain/1
  Gain/1 -> Add/1
  Gain1/1 -> Add/2
  Constant1/1 -> Math Function2/2
  [t] -> Math Function2/1
  Math Function2/1 -> Gain1/1
  Add/1 -> Gain6/1
  Gain2/1 -> Add1/1
  [t] -> Math Function4/1
  Math Function4/1 -> Gain3/1
  Gain3/1 -> Add1/2
  Constant3/1 -> Math Function4/2
  Constant2/1 -> Math Function3/2
  [t] -> Math Function3/1
  Math Function3/1 -> Gain2/1
  Add1/1 -> Gain7/1
  Gain4/1 -> Add2/1
  Gain5/1 -> Add2/2
  Constant4/1 -> Math Function5/2
  [t] -> Math Function5/1
  Math Function5/1 -> Gain4/1
  [t] -> Gain5/1
  Add2/1 -> Gain8/1
  Gain8/1 -> acc1_input/1
  Gain7/1 -> velocity1_input/1
  Gain6/1 -> Theta1_input/1

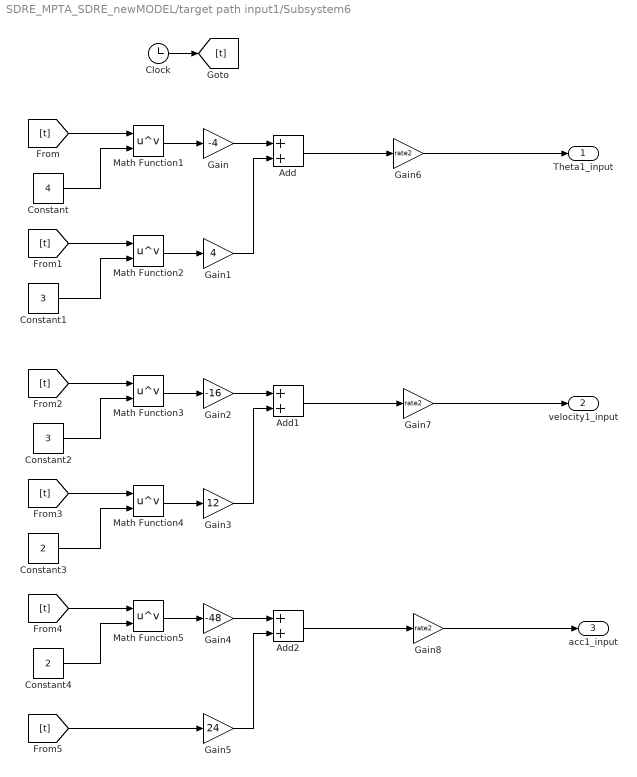
== system SDRE_MPTA_SDRE_newMODEL/target path input1/Subsystem6 ==
  Add : Sum
  Add1 : Sum
  Add2 : Sum
  Clock : Clock
  Constant : Constant  Value=4
  Constant1 : Constant  Value=3
  Constant2 : Constant  Value=3
  Constant3 : Constant  Value=2
  Constant4 : Constant  Value=2
  Gain : Gain  Gain=-4
  Gain1 : Gain  Gain=4
  Gain2 : Gain  Gain=-16
  Gain3 : Gain  Gain=12
  Gain4 : Gain  Gain=-48
  Gain5 : Gain  Gain=24
  Gain6 : Gain  Gain=rate2
  Gain7 : Gain  Gain=rate2
  Gain8 : Gain  Gain=rate2
  Math Function{1..5} (5 alike) : Math  Operator=pow
  Theta1_input : Outport
  velocity1_input : Outport  Port=2
  acc1_input : Outport  Port=3
  wires:
  Clock/1 -> [t]
  [t] -> Math Function1/1
  Constant/1 -> Math Function1/2
  Math Function1/1 -> Gain/1
  Gain/1 -> Add/1
  Gain1/1 -> Add/2
  Constant1/1 -> Math Function2/2
  [t] -> Math Function2/1
  Math Function2/1 -> Gain1/1
  Add/1 -> Gain6/1
  Gain2/1 -> Add1/1
  [t] -> Math Function4/1
  Math Function4/1 -> Gain3/1
  Gain3/1 -> Add1/2
  Constant3/1 -> Math Function4/2
  Constant2/1 -> Math Function3/2
  [t] -> Math Function3/1
  Math Function3/1 -> Gain2/1
  Add1/1 -> Gain7/1
  Gain4/1 -> Add2/1
  Gain5/1 -> Add2/2
  Constant4/1 -> Math Function5/2
  [t] -> Math Function5/1
  Math Function5/1 -> Gain4/1
  [t] -> Gain5/1
  Add2/1 -> Gain8/1
  Gain6/1 -> Theta1_input/1
  Gain7/1 -> velocity1_input/1
  Gain8/1 -> acc1_input/1

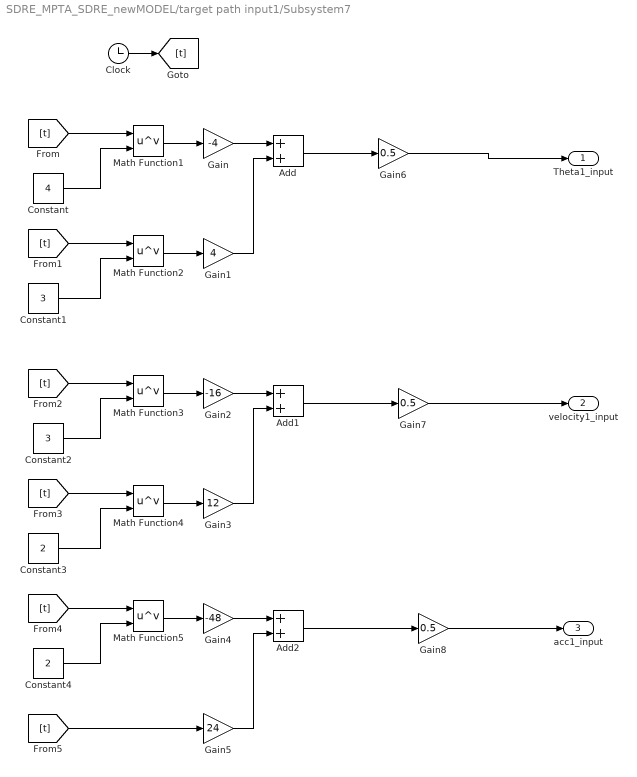
== system SDRE_MPTA_SDRE_newMODEL/target path input1/Subsystem7 ==
  Add : Sum
  Add1 : Sum
  Add2 : Sum
  Clock : Clock
  Constant : Constant  Value=4
  Constant1 : Constant  Value=3
  Constant2 : Constant  Value=3
  Constant3 : Constant  Value=2
  Constant4 : Constant  Value=2
  Gain : Gain  Gain=-4
  Gain1 : Gain  Gain=4
  Gain2 : Gain  Gain=-16
  Gain3 : Gain  Gain=12
  Gain4 : Gain  Gain=-48
  Gain5 : Gain  Gain=24
  Gain6 : Gain  Gain=0.5
  Gain7 : Gain  Gain=0.5
  Gain8 : Gain  Gain=0.5
  Math Function{1..5} (5 alike) : Math  Operator=pow
  Theta1_input : Outport
  velocity1_input : Outport  Port=2
  acc1_input : Outport  Port=3
  wires:
  Clock/1 -> [t]
  [t] -> Math Function1/1
  Constant/1 -> Math Function1/2
  Math Function1/1 -> Gain/1
  Gain/1 -> Add/1
  Gain1/1 -> Add/2
  Constant1/1 -> Math Function2/2
  [t] -> Math Function2/1
  Math Function2/1 -> Gain1/1
  Add/1 -> Gain6/1
  Gain2/1 -> Add1/1
  [t] -> Math Function4/1
  Math Function4/1 -> Gain3/1
  Gain3/1 -> Add1/2
  Constant3/1 -> Math Function4/2
  Constant2/1 -> Math Function3/2
  [t] -> Math Function3/1
  Math Function3/1 -> Gain2/1
  Add1/1 -> Gain7/1
  Gain4/1 -> Add2/1
  Gain5/1 -> Add2/2
  Constant4/1 -> Math Function5/2
  [t] -> Math Function5/1
  Math Function5/1 -> Gain4/1
  [t] -> Gain5/1
  Add2/1 -> Gain8/1
  Gain6/1 -> Theta1_input/1
  Gain7/1 -> velocity1_input/1
  Gain8/1 -> acc1_input/1

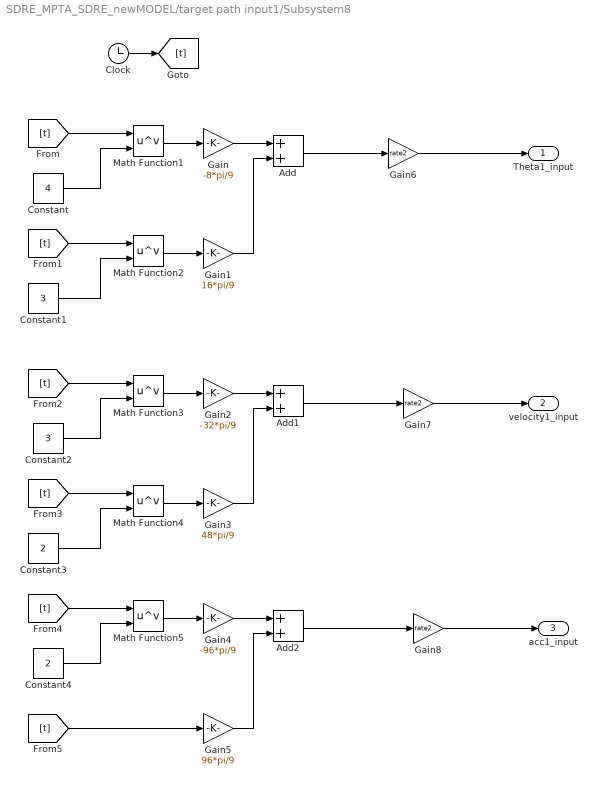
== system SDRE_MPTA_SDRE_newMODEL/target path input1/Subsystem8 ==
  Add : Sum
  Add1 : Sum
  Add2 : Sum
  Clock : Clock
  Constant : Constant  Value=4
  Constant1 : Constant  Value=3
  Constant2 : Constant  Value=3
  Constant3 : Constant  Value=2
  Constant4 : Constant  Value=2
  Gain : Gain  Gain=-8*pi/9
  Gain1 : Gain  Gain=16*pi/9
  Gain2 : Gain  Gain=-32*pi/9
  Gain3 : Gain  Gain=48*pi/9
  Gain4 : Gain  Gain=-96*pi/9
  Gain5 : Gain  Gain=96*pi/9
  Gain6 : Gain  Gain=rate2
  Gain7 : Gain  Gain=rate2
  Gain8 : Gain  Gain=rate2
  Math Function{1..5} (5 alike) : Math  Operator=pow
  Theta1_input : Outport
  velocity1_input : Outport  Port=2
  acc1_input : Outport  Port=3
  wires:
  Clock/1 -> [t]
  [t] -> Math Function1/1
  Constant/1 -> Math Function1/2
  Math Function1/1 -> Gain/1
  Gain/1 -> Add/1
  Gain1/1 -> Add/2
  Constant1/1 -> Math Function2/2
  [t] -> Math Function2/1
  Math Function2/1 -> Gain1/1
  Add/1 -> Gain6/1
  Gain2/1 -> Add1/1
  [t] -> Math Function4/1
  Math Function4/1 -> Gain3/1
  Gain3/1 -> Add1/2
  Constant3/1 -> Math Function4/2
  Constant2/1 -> Math Function3/2
  [t] -> Math Function3/1
  Math Function3/1 -> Gain2/1
  Add1/1 -> Gain7/1
  Gain4/1 -> Add2/1
  Gain5/1 -> Add2/2
  Constant4/1 -> Math Function5/2
  [t] -> Math Function5/1
  Math Function5/1 -> Gain4/1
  [t] -> Gain5/1
  Add2/1 -> Gain8/1
  Gain8/1 -> acc1_input/1
  Gain7/1 -> velocity1_input/1
  Gain6/1 -> Theta1_input/1

== system SDRE_MPTA_SDRE_newMODEL/nomal1/toq to voltageABC6/Inverse Clarke Transform ==
  note: Inverse Clarke Transform
  note: Converts direct axis (alpha) component and the quadrature axis (beta) component to balanced three-phase quantities
      | The alpha and beta components are dependent on time and speed.
  Alpha : Inport
  Beta : Inport  Port=2
  Add : Sum  Inputs=-+  OutDataTypeStr=Inherit: Same as first input
  Add1 : Sum  Inputs=--  OutDataTypeStr=Inherit: Same as first input
  Gain : Gain  Gain=1/2
  Gain1 : Gain  Gain=sqrt(3)/2
  Mux : Mux  Inputs=3
  ABC : Outport  VectorParamsAs1DForOutWhenUnconnected=off
  wires:
  Beta/1 -> Gain1/1
  Mux/1 -> ABC/1
  Alpha/1 -> Mux/1, Gain/1
  Add1/1 -> Mux/3
  Gain1/1 -> Add1/2, Add/2
  Gain/1 -> Add1/1, Add/1
  Add/1 -> Mux/2

== system SDRE_MPTA_SDRE_newMODEL/nomal1/toq to voltageABC6/Inverse Park Transform ==
  note: Converts orthogonal rotating reference frame (dq) to two-phase orthogonal stationary reference frame (alpha, beta)
  note: Inverse Park Transform
  D : Inport
  Q : Inport  Port=2
  Sin_Coefficient : Inport  Port=3
  Cos_Coefficient : Inport  Port=4
  Add1 : Sum  Inputs=+-  OutDataTypeStr=Inherit: Same as first input
  Add2 : Sum  OutDataTypeStr=Inherit: Same as first input
  Cos_Coefficient_1 : InportShadow  Port=4
  Product{1..4} (4 alike) : Product  RndMeth=Simplest
  Sin_Coefficient_1 : InportShadow  Port=3
  Alpha : Outport  VectorParamsAs1DForOutWhenUnconnected=off
  Beta : Outport  Port=2  VectorParamsAs1DForOutWhenUnconnected=off
  wires:
  Sin_Coefficient_1/1 -> Product3/2
  Product2/1 -> Add1/2
  Cos_Coefficient_1/1 -> Product4/2
  Add2/1 -> Beta/1
  Product3/1 -> Add2/1
  Add1/1 -> Alpha/1
  Product1/1 -> Add1/1
  Product4/1 -> Add2/2
  Sin_Coefficient/1 -> Product2/2
  D/1 -> Product3/1, Product1/1
  Q/1 -> Product2/1, Product4/1
  Cos_Coefficient/1 -> Product1/2

== system SDRE_MPTA_SDRE_newMODEL/nomal1/toq to voltageABC6/Subsystem ==
  In1 : Inport
  Bus Selector : BusSelector  OutputSignals=Rotor speed wm (rad/s),Stator current is_d (A),Stator current is_q (A)
  Divide5 : Product  Commented=on  Inputs=*/
  Gain1 : Gain  Gain=Polepairs
  Rate_Transition2 : RateTransition  Integrity=off  Deterministic=off
  Rate_Transition3 : RateTransition  Integrity=off  Deterministic=off
  Rate_Transition4 : RateTransition  Integrity=off  Deterministic=off
  Scope : Scope
  Subsystem : Subsystem
  rad/s to rpm : Gain  Gain=60/(2*pi)
  Out1 : Outport
  Out2 : Outport  Port=2
  Out3 : Outport  Port=3
  wires:
  Gain1/1 -> rad/s to rpm/1
  rad/s to rpm/1 -> Rate_Transition2/1
  Rate_Transition4/1 -> Subsystem/2(In2), Subsystem/3(In3), Out3/1
  Bus Selector/1 -> Gain1/1  "<Rotor speed wm (rad/s)>"
  Bus Selector/3 -> Rate_Transition4/1  "<Stator current is_q (A)>"
  Bus Selector/2 -> Rate_Transition3/1  "<Stator current is_d (A)>"
  In1/1 -> Bus Selector/1
  Rate_Transition3/1 -> Subsystem/1(In1), Out1/1
  Rate_Transition2/1 -> Out2/1
  Subsystem/1(Out1) -> Scope/1

== system SDRE_MPTA_SDRE_newMODEL/nomal1/toq to voltageABC6/Subsystem1 ==
  In1 : Inport
  Rate_Transition1 : RateTransition  Integrity=off
  Out1 : Outport  VectorParamsAs1DForOutWhenUnconnected=off
  wires:
  In1/1 -> Rate_Transition1/1
  Rate_Transition1/1 -> Out1/1

== system SDRE_MPTA_SDRE_newMODEL/nomal1/toq to voltageABC6/Subsystem2 ==
  In1 : Inport
  In2 : Inport  Port=2
  In3 : Inport  Port=3
  Derivative : Derivative
  Derivative1 : Derivative
  Gain : Gain  Gain=Polepairs
  ras/s to rev/min : Gain  Gain=60/(2*pi)
  Out1 : Outport
  Out2 : Outport  Port=2
  Out3 : Outport  Port=3
  Out4 : Outport  Port=4
  Out5 : Outport  Port=5
  wires:
  In2/1 -> Derivative/1, Out2/1
  In3/1 -> Derivative1/1, Out3/1
  In1/1 -> Gain/1
  Derivative/1 -> Out4/1
  Derivative1/1 -> Out5/1
  Gain/1 -> ras/s to rev/min/1
  ras/s to rev/min/1 -> Out1/1

== system SDRE_MPTA_SDRE_newMODEL/nomal1/toq to voltageABC6/ideal_voltage_source1 ==
  note: PWM Peripheral And Inverter
  Vabc : Inport
  Controlled_Voltage_Source1 : spsControlledVoltageSourceLib/Controlled Voltage Source  Initialize=off  Source_Type=DC  Amplitude=12  Phase=0  Frequency=0  Measurements=None
  Controlled_Voltage_Source2 : spsControlledVoltageSourceLib/Controlled Voltage Source  Initialize=off  Source_Type=DC  Amplitude=12  Phase=0  Frequency=0  Measurements=None
  Controlled_Voltage_Source3 : spsControlledVoltageSourceLib/Controlled Voltage Source  Initialize=off  Source_Type=DC  Amplitude=12  Phase=0  Frequency=0  Measurements=None
  Ground2 : spsGroundLib/Ground  LConnTagsString=a
  Selector3 : Selector  InputPortWidth=3  IndexOptions=Index vector (dialog)  Indices=[1]  OutputSizes=1
  Selector4 : Selector  InputPortWidth=3  IndexOptions=Index vector (dialog)  Indices=2  OutputSizes=1
  Selector5 : Selector  InputPortWidth=3  IndexOptions=Index vector (dialog)  Indices=3  OutputSizes=1
  A : PMIOPort  Tag=PMCPort  Side=Right
  B : PMIOPort  Tag=PMCPort  Port=2  Side=Right
  C : PMIOPort  Tag=PMCPort  Port=3  Side=Right
  wires:
  Vabc/1 -> Selector4/1, Selector5/1, Selector3/1
  Selector5/1 -> Controlled_Voltage_Source3/1
  Selector4/1 -> Controlled_Voltage_Source2/1
  Selector3/1 -> Controlled_Voltage_Source1/1
  connections:
  C/RConn1 -- Controlled_Voltage_Source3/RConn1
  B/RConn1 -- Controlled_Voltage_Source2/RConn1
  A/RConn1 -- Controlled_Voltage_Source1/RConn1
  Controlled_Voltage_Source3/LConn1 -- Controlled_Voltage_Source1/LConn1 -- Controlled_Voltage_Source2/LConn1 -- Ground2/LConn1

== system SDRE_MPTA_SDRE_newMODEL/nomal3/toq to voltageABC/If Action Subsystem ==
  In1 : Inport
  Action Port : ActionPort  ActionPortLabel=else
  Out1 : Outport
  wires:
  In1/1 -> Out1/1

== system SDRE_MPTA_SDRE_newMODEL/nomal3/toq to voltageABC/If Action Subsystem1 ==
  In1 : Inport
  Action Port : ActionPort  ActionPortLabel=if((u1)< 1e-10)
  Out1 : Outport
  wires:
  In1/1 -> Out1/1

== system SDRE_MPTA_SDRE_newMODEL/nomal3/toq to voltageABC/If Action Subsystem2 ==
  In1 : Inport
  Action Port : ActionPort  ActionPortLabel=else
  Out1 : Outport
  wires:
  In1/1 -> Out1/1

== system SDRE_MPTA_SDRE_newMODEL/nomal3/toq to voltageABC/If Action Subsystem3 ==
  In1 : Inport
  Action Port : ActionPort  ActionPortLabel=if(u1 < 1e-10)
  Out1 : Outport
  wires:
  In1/1 -> Out1/1

== system SDRE_MPTA_SDRE_newMODEL/nomal3/toq to voltageABC/Subsystem ==
  In1 : Inport
  In2 : Inport  Port=2
  In3 : Inport  Port=3
  Add : Sum
  Constant : Constant  Value=3*Polepairs/2
  Constant1 : Constant  Value=Lambda_m
  Gain : Gain  Gain=Ldq
  Product : Product
  Product1 : Product
  Product2 : Product
  Out1 : Outport
  wires:
  Product1/1 -> Add/2
  Product2/1 -> Gain/1
  Product/1 -> Out1/1
  Constant/1 -> Product/2
  In3/1 -> Product2/1
  Add/1 -> Product/1
  Gain/1 -> Add/1
  Constant1/1 -> Product1/2
  In1/1 -> Product2/2
  In2/1 -> Product1/1

== system SDRE_MPTA_SDRE_newMODEL/nomal3/toq to voltageABC6/Inverse Clarke Transform ==
  note: Inverse Clarke Transform
  note: Converts direct axis (alpha) component and the quadrature axis (beta) component to balanced three-phase quantities
      | The alpha and beta components are dependent on time and speed.
  Alpha : Inport
  Beta : Inport  Port=2
  Add : Sum  Inputs=-+  OutDataTypeStr=Inherit: Same as first input
  Add1 : Sum  Inputs=--  OutDataTypeStr=Inherit: Same as first input
  Gain : Gain  Gain=1/2
  Gain1 : Gain  Gain=sqrt(3)/2
  Mux : Mux  Inputs=3
  ABC : Outport  VectorParamsAs1DForOutWhenUnconnected=off
  wires:
  Beta/1 -> Gain1/1
  Mux/1 -> ABC/1
  Alpha/1 -> Mux/1, Gain/1
  Add1/1 -> Mux/3
  Gain1/1 -> Add1/2, Add/2
  Gain/1 -> Add1/1, Add/1
  Add/1 -> Mux/2

== system SDRE_MPTA_SDRE_newMODEL/nomal3/toq to voltageABC6/Inverse Park Transform ==
  note: Converts orthogonal rotating reference frame (dq) to two-phase orthogonal stationary reference frame (alpha, beta)
  note: Inverse Park Transform
  D : Inport
  Q : Inport  Port=2
  Sin_Coefficient : Inport  Port=3
  Cos_Coefficient : Inport  Port=4
  Add1 : Sum  Inputs=+-  OutDataTypeStr=Inherit: Same as first input
  Add2 : Sum  OutDataTypeStr=Inherit: Same as first input
  Cos_Coefficient_1 : InportShadow  Port=4
  Product{1..4} (4 alike) : Product  RndMeth=Simplest
  Sin_Coefficient_1 : InportShadow  Port=3
  Alpha : Outport  VectorParamsAs1DForOutWhenUnconnected=off
  Beta : Outport  Port=2  VectorParamsAs1DForOutWhenUnconnected=off
  wires:
  Sin_Coefficient_1/1 -> Product3/2
  Product2/1 -> Add1/2
  Cos_Coefficient_1/1 -> Product4/2
  Add2/1 -> Beta/1
  Product3/1 -> Add2/1
  Add1/1 -> Alpha/1
  Product1/1 -> Add1/1
  Product4/1 -> Add2/2
  Sin_Coefficient/1 -> Product2/2
  D/1 -> Product3/1, Product1/1
  Q/1 -> Product2/1, Product4/1
  Cos_Coefficient/1 -> Product1/2

== system SDRE_MPTA_SDRE_newMODEL/nomal3/toq to voltageABC6/Subsystem ==
  In1 : Inport
  Bus Selector : BusSelector  OutputSignals=Rotor speed wm (rad/s),Stator current is_d (A),Stator current is_q (A)
  Divide5 : Product  Commented=on  Inputs=*/
  Gain1 : Gain  Gain=Polepairs
  Rate_Transition2 : RateTransition  Integrity=off  Deterministic=off
  Rate_Transition3 : RateTransition  Integrity=off  Deterministic=off
  Rate_Transition4 : RateTransition  Integrity=off  Deterministic=off
  Scope : Scope
  Subsystem : Subsystem
  rad/s to rpm : Gain  Gain=60/(2*pi)
  Out1 : Outport
  Out2 : Outport  Port=2
  Out3 : Outport  Port=3
  wires:
  Gain1/1 -> rad/s to rpm/1
  rad/s to rpm/1 -> Rate_Transition2/1
  Rate_Transition4/1 -> Subsystem/2(In2), Subsystem/3(In3), Out3/1
  Bus Selector/1 -> Gain1/1  "<Rotor speed wm (rad/s)>"
  Bus Selector/3 -> Rate_Transition4/1  "<Stator current is_q (A)>"
  Bus Selector/2 -> Rate_Transition3/1  "<Stator current is_d (A)>"
  In1/1 -> Bus Selector/1
  Rate_Transition3/1 -> Subsystem/1(In1), Out1/1
  Rate_Transition2/1 -> Out2/1
  Subsystem/1(Out1) -> Scope/1

== system SDRE_MPTA_SDRE_newMODEL/nomal3/toq to voltageABC6/Subsystem1 ==
  In1 : Inport
  Rate_Transition1 : RateTransition  Integrity=off
  Out1 : Outport  VectorParamsAs1DForOutWhenUnconnected=off
  wires:
  In1/1 -> Rate_Transition1/1
  Rate_Transition1/1 -> Out1/1

== system SDRE_MPTA_SDRE_newMODEL/nomal3/toq to voltageABC6/Subsystem2 ==
  In1 : Inport
  In2 : Inport  Port=2
  In3 : Inport  Port=3
  Derivative : Derivative
  Derivative1 : Derivative
  Gain : Gain  Gain=Polepairs
  ras/s to rev/min : Gain  Gain=60/(2*pi)
  Out1 : Outport
  Out2 : Outport  Port=2
  Out3 : Outport  Port=3
  Out4 : Outport  Port=4
  Out5 : Outport  Port=5
  wires:
  In2/1 -> Derivative/1, Out2/1
  In3/1 -> Derivative1/1, Out3/1
  In1/1 -> Gain/1
  Derivative/1 -> Out4/1
  Derivative1/1 -> Out5/1
  Gain/1 -> ras/s to rev/min/1
  ras/s to rev/min/1 -> Out1/1

== system SDRE_MPTA_SDRE_newMODEL/nomal3/toq to voltageABC6/ideal_voltage_source1 ==
  note: PWM Peripheral And Inverter
  Vabc : Inport
  Controlled_Voltage_Source1 : spsControlledVoltageSourceLib/Controlled Voltage Source  Initialize=off  Source_Type=DC  Amplitude=12  Phase=0  Frequency=0  Measurements=None
  Controlled_Voltage_Source2 : spsControlledVoltageSourceLib/Controlled Voltage Source  Initialize=off  Source_Type=DC  Amplitude=12  Phase=0  Frequency=0  Measurements=None
  Controlled_Voltage_Source3 : spsControlledVoltageSourceLib/Controlled Voltage Source  Initialize=off  Source_Type=DC  Amplitude=12  Phase=0  Frequency=0  Measurements=None
  Ground2 : spsGroundLib/Ground  LConnTagsString=a
  Selector3 : Selector  InputPortWidth=3  IndexOptions=Index vector (dialog)  Indices=[1]  OutputSizes=1
  Selector4 : Selector  InputPortWidth=3  IndexOptions=Index vector (dialog)  Indices=2  OutputSizes=1
  Selector5 : Selector  InputPortWidth=3  IndexOptions=Index vector (dialog)  Indices=3  OutputSizes=1
  A : PMIOPort  Tag=PMCPort  Side=Right
  B : PMIOPort  Tag=PMCPort  Port=2  Side=Right
  C : PMIOPort  Tag=PMCPort  Port=3  Side=Right
  wires:
  Vabc/1 -> Selector4/1, Selector5/1, Selector3/1
  Selector5/1 -> Controlled_Voltage_Source3/1
  Selector4/1 -> Controlled_Voltage_Source2/1
  Selector3/1 -> Controlled_Voltage_Source1/1
  connections:
  C/RConn1 -- Controlled_Voltage_Source3/RConn1
  B/RConn1 -- Controlled_Voltage_Source2/RConn1
  A/RConn1 -- Controlled_Voltage_Source1/RConn1
  Controlled_Voltage_Source3/LConn1 -- Controlled_Voltage_Source1/LConn1 -- Controlled_Voltage_Source2/LConn1 -- Ground2/LConn1

== system SDRE_MPTA_SDRE_newMODEL/nomal1/toq to voltageABC6/Subsystem/Subsystem ==
  In1 : Inport
  In2 : Inport  Port=2
  In3 : Inport  Port=3
  Add : Sum
  Constant : Constant  Value=3*Polepairs/2
  Constant1 : Constant  Value=Lambda_m
  Gain : Gain  Gain=Ldq
  Product : Product
  Product1 : Product
  Product2 : Product
  Out1 : Outport
  wires:
  Product1/1 -> Add/2
  Product2/1 -> Gain/1
  Product/1 -> Out1/1
  Constant/1 -> Product/2
  In3/1 -> Product2/1
  Add/1 -> Product/1
  Gain/1 -> Add/1
  Constant1/1 -> Product1/2
  In1/1 -> Product2/2
  In2/1 -> Product1/1

== system SDRE_MPTA_SDRE_newMODEL/nomal3/toq to voltageABC6/Subsystem/Subsystem ==
  In1 : Inport
  In2 : Inport  Port=2
  In3 : Inport  Port=3
  Add : Sum
  Constant : Constant  Value=3*Polepairs/2
  Constant1 : Constant  Value=Lambda_m
  Gain : Gain  Gain=Ldq
  Product : Product
  Product1 : Product
  Product2 : Product
  Out1 : Outport
  wires:
  Product1/1 -> Add/2
  Product2/1 -> Gain/1
  Product/1 -> Out1/1
  Constant/1 -> Product/2
  In3/1 -> Product2/1
  Add/1 -> Product/1
  Gain/1 -> Add/1
  Constant1/1 -> Product1/2
  In1/1 -> Product2/2
  In2/1 -> Product1/1
